simulink model "openMHA_test_FFT_to_gain"  (R2020b)
settings: Solver=VariableStepAuto  StartTime=0.0  StopTime=stop_time  RelTol=1e-3
InitFcn:
  | test_FFT_to_gain_init
StopFcn:
  | test_FFT_to_gain_stop
values from neighbouring files (symbols this model uses):
  accum_delay = max(band_sizes)    [test_FFT_to_gain_init.m]
  accum_delay_memory_size = 2^accum_delay_memory    [test_FFT_to_gain_init.m]
  band_edges = [band_edges mirrored_band_edges]    [test_FFT_to_gain_init.m]
  buf_a = 65.*ones(num_bands,1)    [test_FFT_to_gain_init.m]    (also in test_db_ar_gaintable_init.m)
  buf_r = 65.*ones(num_bands,1)    [test_FFT_to_gain_init.m]    (also in test_db_ar_gaintable_init.m)
  delay_memory_size = 2^system_delay_memory    [test_FFT_to_gain_init.m]
  FFTsize = 256    [test_FFT_to_gain_init.m]    (also in test_db_ar_gaintable_init.m)
  gainapp_dp_memory = log2(num_bands) + 1    [test_FFT_to_gain_init.m]
  num_bands = 8    [test_FFT_to_gain_init.m]    (also in test_db_ar_gaintable_init.m = 2)
  num_bins = FFTsize/2 + 1    (= 129)    [test_FFT_to_gain_init.m]    (also in test_db_ar_gaintable_init.m)
  system_delay = 70    [calculate_gainapp_test_signals.m]    (also in test_FFT_to_gain_init.m = gain_delay + accum_delay)
  table_length = length(gtdata)    [test_FFT_to_gain_init.m]    (also in test_db_ar_gaintable_init.m)
  X_high = 93    [test_FFT_to_gain_init.m]    (also in test_db_ar_gaintable_init.m)
undefined symbols (not defined in the file or in its folder): xIn
libraries: dspsrcs4 x9, hdlsllib x8, simulink x8, FPGA_Open_Speech_Tools x5
(part 1 of 2)
settings Model: SnapshotBufferSize=20  Creator=t96f346  LastModifiedBy=t96f346

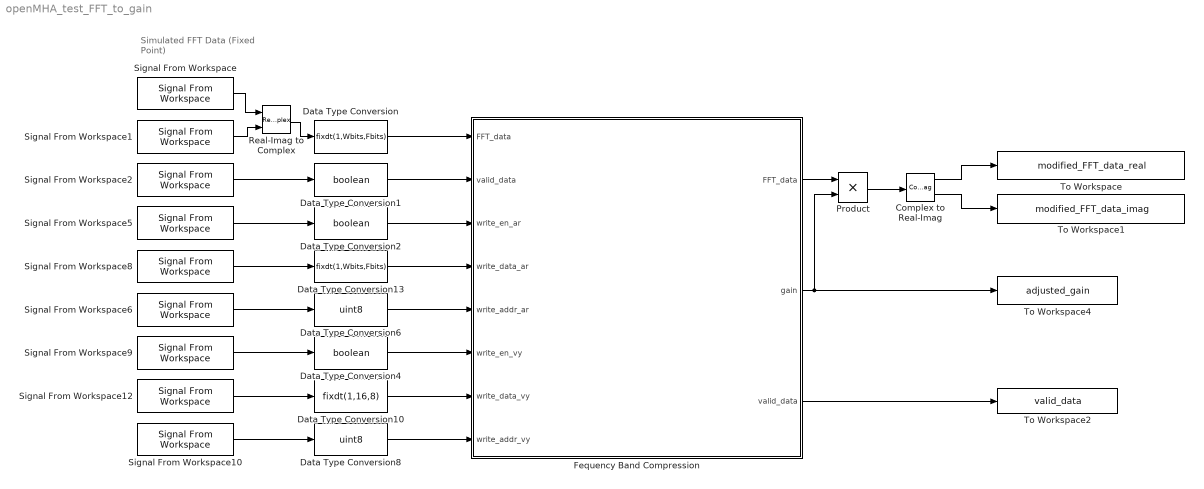
== system openMHA_test_FFT_to_gain ==
  note: Simulated FFT Data
      | (Fixed Point)
  Complex to Real-Imag : ComplexToRealImag
  Data Type Conversion : DataTypeConversion  OutDataTypeStr=fixdt(1,Wbits,Fbits)
  Data Type Conversion1 : DataTypeConversion  OutDataTypeStr=boolean
  Data Type Conversion10 : DataTypeConversion  OutDataTypeStr=fixdt(1,16,8)
  Data Type Conversion13 : DataTypeConversion  OutDataTypeStr=fixdt(1,Wbits,Fbits)
  Data Type Conversion2 : DataTypeConversion  OutDataTypeStr=boolean
  Data Type Conversion4 : DataTypeConversion  OutDataTypeStr=boolean
  Data Type Conversion6 : DataTypeConversion  OutDataTypeStr=uint8
  Data Type Conversion8 : DataTypeConversion  OutDataTypeStr=uint8
  Fequency Band Compression : Subsystem
  Product : Product  OutDataTypeStr=fixdt(1,Wbits,Fbits)
  Real-Imag to Complex : RealImagToComplex
  Signal From Workspace : dspsrcs4/Signal From Workspace  X=FFT_data_real  Ts=1  nsamps=1  OutputAfterFinalValue=Setting to zero  ignoreOrWarnInputAndFrameLengths=off  OutputFrames=off
  Signal From Workspace1 : dspsrcs4/Signal From Workspace  X=FFT_data_imag  Ts=1  nsamps=1  OutputAfterFinalValue=Setting to zero  ignoreOrWarnInputAndFrameLengths=off  OutputFrames=off
  Signal From Workspace10 : dspsrcs4/Signal From Workspace  X=write_addr_vy  Ts=1  nsamps=1  OutputAfterFinalValue=Setting to zero  ignoreOrWarnInputAndFrameLengths=off  OutputFrames=off
  Signal From Workspace12 : dspsrcs4/Signal From Workspace  X=write_data_vy  Ts=1  nsamps=1  OutputAfterFinalValue=Setting to zero  ignoreOrWarnInputAndFrameLengths=off  OutputFrames=off
  Signal From Workspace2 : dspsrcs4/Signal From Workspace  X=valid_data  Ts=1  nsamps=1  OutputAfterFinalValue=Setting to zero  ignoreOrWarnInputAndFrameLengths=off  OutputFrames=off
  Signal From Workspace5 : dspsrcs4/Signal From Workspace  X=write_en_ar  Ts=1  nsamps=1  OutputAfterFinalValue=Setting to zero  ignoreOrWarnInputAndFrameLengths=off  OutputFrames=off
  Signal From Workspace6 : dspsrcs4/Signal From Workspace  X=write_addr_ar  Ts=1  nsamps=1  OutputAfterFinalValue=Setting to zero  ignoreOrWarnInputAndFrameLengths=off  OutputFrames=off
  Signal From Workspace8 : dspsrcs4/Signal From Workspace  X=write_data_ar  Ts=1  nsamps=1  OutputAfterFinalValue=Setting to zero  ignoreOrWarnInputAndFrameLengths=off  OutputFrames=off
  Signal From Workspace9 : dspsrcs4/Signal From Workspace  X=write_en_vy  Ts=1  nsamps=1  OutputAfterFinalValue=Setting to zero  ignoreOrWarnInputAndFrameLengths=off  OutputFrames=off
  To Workspace : ToWorkspace  VariableName=modified_FFT_data_real  SampleTime=-1
      settings: Save2DSignal=2-D array (concatenate along first dimension)
  To Workspace1 : ToWorkspace  VariableName=modified_FFT_data_imag  SampleTime=-1
      settings: Save2DSignal=2-D array (concatenate along first dimension)
  To Workspace2 : ToWorkspace  VariableName=valid_data  SampleTime=-1
      settings: Save2DSignal=2-D array (concatenate along first dimension)
  To Workspace4 : ToWorkspace  VariableName=adjusted_gain  SampleTime=-1
      settings: Save2DSignal=2-D array (concatenate along first dimension)
  wires:
  Real-Imag to Complex/1 -> Data Type Conversion/1
  Signal From Workspace1/1 -> Real-Imag to Complex/2
  Signal From Workspace/1 -> Real-Imag to Complex/1
  Product/1 -> Complex to Real-Imag/1
  Complex to Real-Imag/2 -> To Workspace1/1
  Complex to Real-Imag/1 -> To Workspace/1
  Data Type Conversion/1 -> Fequency Band Compression/1(FFT_data)
  Signal From Workspace2/1 -> Data Type Conversion1/1
  Signal From Workspace12/1 -> Data Type Conversion10/1
  Signal From Workspace8/1 -> Data Type Conversion13/1
  Signal From Workspace10/1 -> Data Type Conversion8/1
  Signal From Workspace9/1 -> Data Type Conversion4/1
  Signal From Workspace6/1 -> Data Type Conversion6/1
  Signal From Workspace5/1 -> Data Type Conversion2/1
  Data Type Conversion2/1 -> Fequency Band Compression/3(write_en_ar)
  Data Type Conversion13/1 -> Fequency Band Compression/4(write_data_ar)
  Data Type Conversion6/1 -> Fequency Band Compression/5(write_addr_ar)
  Data Type Conversion4/1 -> Fequency Band Compression/6(write_en_vy)
  Data Type Conversion10/1 -> Fequency Band Compression/7(write_data_vy)
  Data Type Conversion8/1 -> Fequency Band Compression/8(write_addr_vy)
  Fequency Band Compression/2(gain) -> Product/2, To Workspace4/1
  Data Type Conversion1/1 -> Fequency Band Compression/2(valid_data)
  Fequency Band Compression/1("FFT_data ") -> Product/1
  Fequency Band Compression/3("valid_data ") -> To Workspace2/1

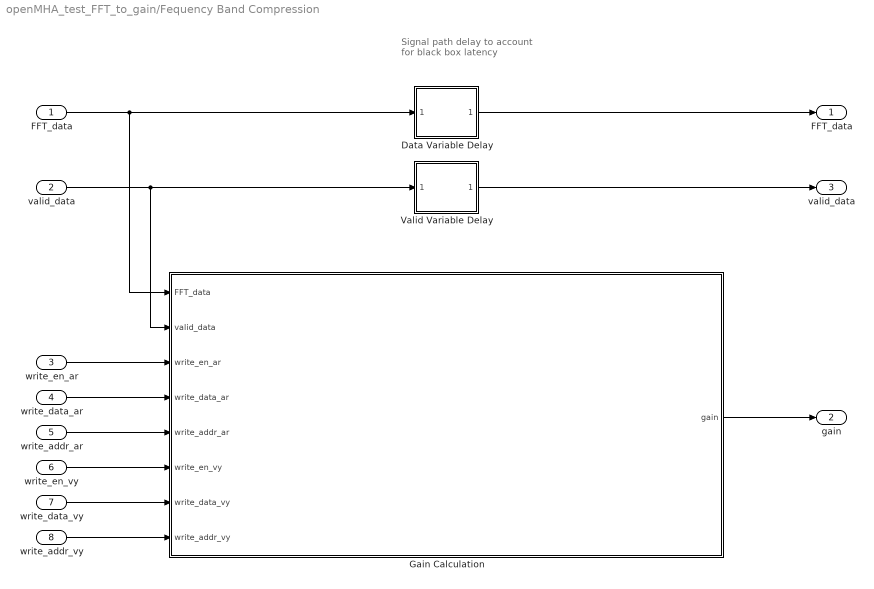
== system openMHA_test_FFT_to_gain/Fequency Band Compression ==
  note: Signal path delay to account for black box latency
  FFT_data : Inport
  valid_data : Inport  Port=2
  write_en_ar : Inport  Port=3
  write_data_ar : Inport  Port=4
  write_addr_ar : Inport  Port=5
  write_en_vy : Inport  Port=6
  write_data_vy : Inport  Port=7
  write_addr_vy : Inport  Port=8
  Data Variable Delay : Subsystem
  Gain Calculation : Subsystem
  Valid Variable Delay : Subsystem
  "FFT_data " : Outport
  gain : Outport  Port=2
  "valid_data " : Outport  Port=3
  wires:
  valid_data/1 -> Gain Calculation/2(valid_data), Valid Variable Delay/1(data_in)
  FFT_data/1 -> Gain Calculation/1(FFT_data), Data Variable Delay/1(data_in)
  Valid Variable Delay/1(rd_dout) -> "valid_data "/1
  Data Variable Delay/1(rd_dout) -> "FFT_data "/1
  write_en_ar/1 -> Gain Calculation/3(write_en_ar)
  write_data_ar/1 -> Gain Calculation/4(write_data_ar)
  write_addr_ar/1 -> Gain Calculation/5(write_addr_ar)
  write_en_vy/1 -> Gain Calculation/6(write_en_vy)
  write_data_vy/1 -> Gain Calculation/7(write_data_vy)
  write_addr_vy/1 -> Gain Calculation/8(write_addr_vy)
  Gain Calculation/1("gain ") -> gain/1

== system openMHA_test_FFT_to_gain/Fequency Band Compression/Data Variable Delay ==
  data_in : Inport
  Constant : Constant  Value=system_delay  OutDataTypeStr=uint8  SampleTime=-1
  Constant2 : Constant  OutDataTypeStr=Inherit: Inherit via back propagation  SampleTime=-1
  integer delay DPRAM : hdlsllib/HDL RAMs/Simple Dual Port RAM  ram_size=system_delay_memory
      settings: SourceProductBaseCode=SL
  read address generator : Subsystem
  write address generator : hdlsllib/Sources/HDL Counter  CountType=Count limited  CountInit=0  CountStep=1  CountMax=delay_memory_size - 1  CountFromType=Initial value  CountFrom=0  CountResetPort=off  CountLoadPort=off  CountEnbPort=off  CountDirPort=off  CountDataType=Unsigned  CountWordLen=system_delay_memory  CountFracLen=0  CountSampTime=-1
  rd_dout : Outport
  wires:
  Constant2/1 -> integer delay DPRAM/3
  write address generator/1 -> integer delay DPRAM/2, read address generator/1(write_addr)
  integer delay DPRAM/1 -> rd_dout/1
  Constant/1 -> read address generator/2(delay)
  data_in/1 -> integer delay DPRAM/1
  read address generator/1(read_addr) -> integer delay DPRAM/4

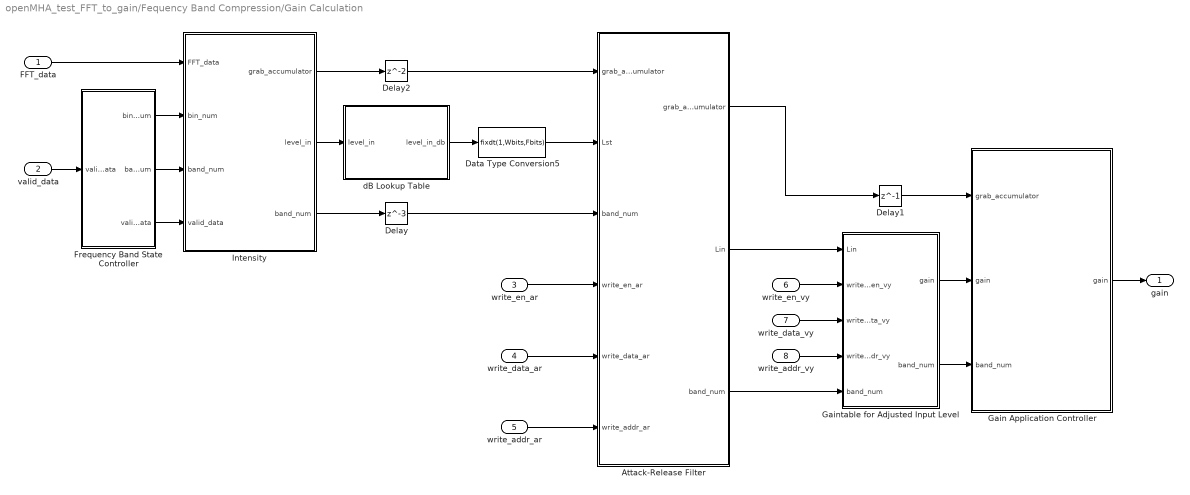
== system openMHA_test_FFT_to_gain/Fequency Band Compression/Gain Calculation ==
  FFT_data : Inport
  valid_data : Inport  Port=2
  write_en_ar : Inport  Port=3
  write_data_ar : Inport  Port=4
  write_addr_ar : Inport  Port=5
  write_en_vy : Inport  Port=6
  write_data_vy : Inport  Port=7
  write_addr_vy : Inport  Port=8
  Attack-Release Filter : Subsystem
  Data Type Conversion5 : DataTypeConversion  OutDataTypeStr=fixdt(1,Wbits,Fbits)
  Delay : Delay  DelayLength=3  InitialCondition=1
  Delay1 : Delay  DelayLength=1  InitialCondition=0
  Delay2 : Delay  InitialCondition=0
  Frequency Band State Controller : Subsystem
  Gain Application Controller : Subsystem
  Gaintable for Adjusted Input Level : Subsystem
  Intensity : Subsystem
  dB Lookup Table : Subsystem
  "gain " : Outport
  wires:
  dB Lookup Table/1(level_in_db) -> Data Type Conversion5/1
  Gaintable for Adjusted Input Level/1(gain) -> Gain Application Controller/2(gain)
  Intensity/1(grab_accumulator) -> Delay2/1
  Delay2/1 -> Attack-Release Filter/1(grab_accumulator)
  write_en_ar/1 -> Attack-Release Filter/4(write_en_ar)
  Frequency Band State Controller/2(band_num) -> Intensity/3(band_num)
  Intensity/3("band_num ") -> Delay/1
  Attack-Release Filter/3("band_num ") -> Gaintable for Adjusted Input Level/5(band_num)
  Delay1/1 -> Gain Application Controller/1(grab_accumulator)
  Delay/1 -> Attack-Release Filter/3(band_num)
  Attack-Release Filter/2(Lin) -> Gaintable for Adjusted Input Level/1(Lin)
  Frequency Band State Controller/1(bin_num) -> Intensity/2(bin_num)
  Gaintable for Adjusted Input Level/2("band_num ") -> Gain Application Controller/3(band_num)
  Data Type Conversion5/1 -> Attack-Release Filter/2(Lst)
  FFT_data/1 -> Intensity/1(FFT_data)
  Intensity/2(level_in) -> dB Lookup Table/1(level_in)
  write_addr_ar/1 -> Attack-Release Filter/6(write_addr_ar)
  valid_data/1 -> Frequency Band State Controller/1(valid_data)
  write_data_ar/1 -> Attack-Release Filter/5(write_data_ar)
  Gain Application Controller/1("gain ") -> "gain "/1
  Attack-Release Filter/1("grab_accumulator ") -> Delay1/1
  write_en_vy/1 -> Gaintable for Adjusted Input Level/2(write_en_vy)
  write_addr_vy/1 -> Gaintable for Adjusted Input Level/4(write_addr_vy)
  write_data_vy/1 -> Gaintable for Adjusted Input Level/3(write_data_vy)
  Frequency Band State Controller/3("valid_data ") -> Intensity/4("valid_data ")

== system openMHA_test_FFT_to_gain/Fequency Band Compression/Valid Variable Delay ==
  data_in : Inport
  Constant : Constant  Value=system_delay  OutDataTypeStr=uint8  SampleTime=-1
  Constant2 : Constant  OutDataTypeStr=Inherit: Inherit via back propagation  SampleTime=-1
  integer delay DPRAM : hdlsllib/HDL RAMs/Simple Dual Port RAM  ram_size=system_delay_memory
      settings: SourceProductBaseCode=SL
  read address generator : Subsystem
  write address generator : hdlsllib/Sources/HDL Counter  CountType=Count limited  CountInit=0  CountStep=1  CountMax=delay_memory_size - 1  CountFromType=Initial value  CountFrom=0  CountResetPort=off  CountLoadPort=off  CountEnbPort=off  CountDirPort=off  CountDataType=Unsigned  CountWordLen=system_delay_memory  CountFracLen=0  CountSampTime=-1
  rd_dout : Outport
  wires:
  Constant2/1 -> integer delay DPRAM/3
  write address generator/1 -> integer delay DPRAM/2, read address generator/1(write_addr)
  integer delay DPRAM/1 -> rd_dout/1
  Constant/1 -> read address generator/2(delay)
  data_in/1 -> integer delay DPRAM/1
  read address generator/1(read_addr) -> integer delay DPRAM/4

== system openMHA_test_FFT_to_gain/Fequency Band Compression/Data Variable Delay/read address generator ==
  note: wrap on overflow is the desired behavior
  write_addr : Inport
  delay : Inport  Port=2
  Constant : Constant  Value=delay_memory_size  SampleTime=-1
  Subtract : Sum  Inputs=-++  OutDataTypeStr=Inherit: Inherit via back propagation
  read_addr : Outport  VectorParamsAs1DForOutWhenUnconnected=off
  wires:
  Subtract/1 -> read_addr/1
  write_addr/1 -> Subtract/2
  delay/1 -> Subtract/1
  Constant/1 -> Subtract/3

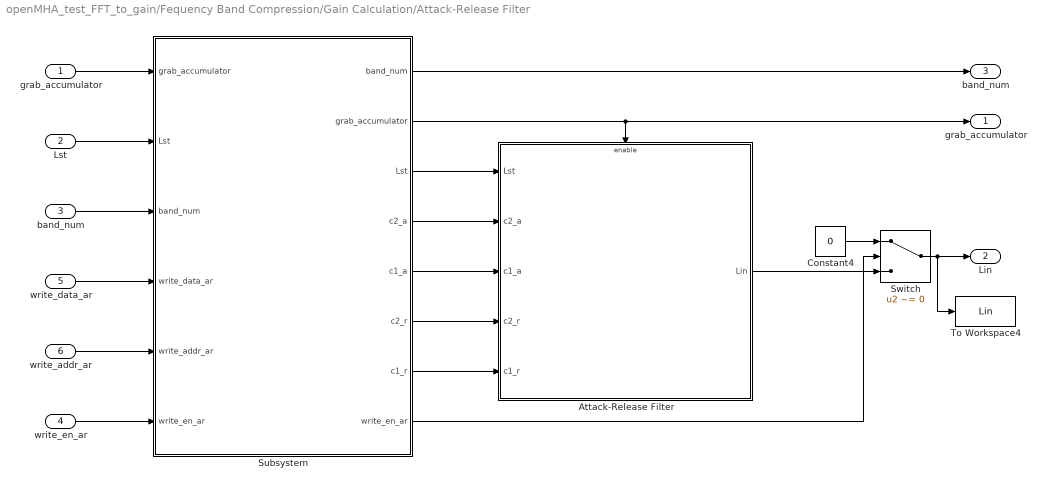
== system openMHA_test_FFT_to_gain/Fequency Band Compression/Gain Calculation/Attack-Release Filter ==
  grab_accumulator : Inport
  Lst : Inport  Port=2
  band_num : Inport  Port=3
  write_en_ar : Inport  Port=4
  write_data_ar : Inport  Port=5
  write_addr_ar : Inport  Port=6
  Attack-Release Filter : Subsystem
  Constant4 : Constant  Value=0  OutDataTypeStr=fixdt(1,Wbits,Fbits)  SampleTime=-1
  Subsystem : Subsystem
  Switch : Switch  Criteria=u2 ~= 0  OutDataTypeStr=fixdt(1,Wbits,Fbits)
  To Workspace4 : ToWorkspace  VariableName=Lin  SampleTime=-1
      settings: Save2DSignal=2-D array (concatenate along first dimension)
  "grab_accumulator " : Outport
  Lin : Outport  Port=2
  "band_num " : Outport  Port=3
  wires:
  Constant4/1 -> Switch/1
  Attack-Release Filter/1(Lin) -> Switch/3
  Switch/1 -> Lin/1, To Workspace4/1
  band_num/1 -> Subsystem/3(band_num)
  Lst/1 -> Subsystem/2(Lst)
  write_data_ar/1 -> Subsystem/4(write_data_ar)
  write_addr_ar/1 -> Subsystem/5(write_addr_ar)
  write_en_ar/1 -> Subsystem/6("write_en_ar ")
  Subsystem/3("Lst ") -> Attack-Release Filter/1(Lst)
  Subsystem/1("band_num ") -> "band_num "/1
  Subsystem/8(write_en_ar) -> Switch/2
  Subsystem/4(c2_a) -> Attack-Release Filter/2(c2_a)
  Subsystem/5(c1_a) -> Attack-Release Filter/3(c1_a)
  Subsystem/6(c2_r) -> Attack-Release Filter/4(c2_r)
  Subsystem/7(c1_r) -> Attack-Release Filter/5(c1_r)
  grab_accumulator/1 -> Subsystem/1(grab_accumulator)
  Subsystem/2("grab_accumulator ") -> "grab_accumulator "/1, Attack-Release Filter/Enable

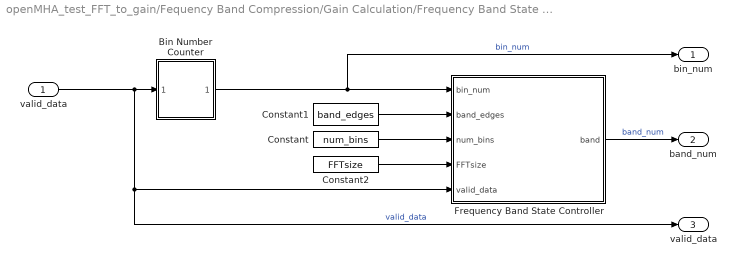
== system openMHA_test_FFT_to_gain/Fequency Band Compression/Gain Calculation/Frequency Band State Controller ==
  valid_data : Inport
  Bin Number Counter : Subsystem
  Constant : Constant  Value=num_bins  SampleTime=-1
  Constant1 : Constant  Value=band_edges  SampleTime=-1
  Constant2 : Constant  Value=FFTsize  SampleTime=-1
  Frequency Band State Controller : MATLAB Function  TreatAsAtomicUnit=on
  bin_num : Outport
  band_num : Outport  Port=2
  "valid_data " : Outport  Port=3
  wires:
  Bin Number Counter/1(bin_num) -> bin_num/1, Frequency Band State Controller/1(bin_num)  "bin_num"
  Constant2/1 -> Frequency Band State Controller/4(FFTsize)
  valid_data/1 -> "valid_data "/1, Frequency Band State Controller/5(valid_data), Bin Number Counter/1(valid_data)  "valid_data"
  Constant/1 -> Frequency Band State Controller/3(num_bins)
  Constant1/1 -> Frequency Band State Controller/2(band_edges)
  Frequency Band State Controller/1(band) -> band_num/1  "band_num"

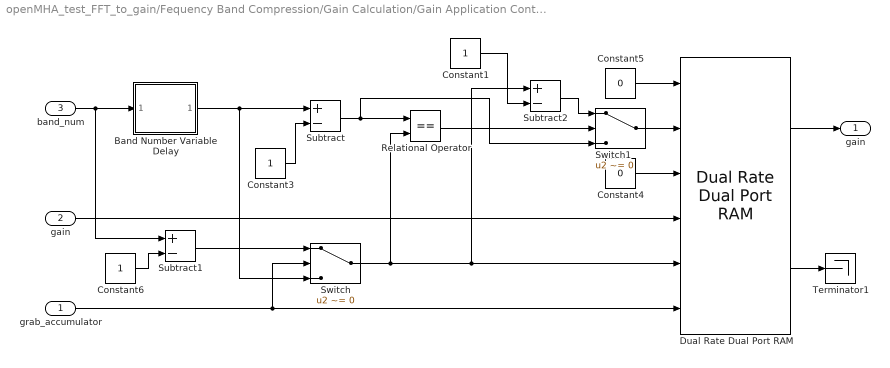
== system openMHA_test_FFT_to_gain/Fequency Band Compression/Gain Calculation/Gain Application Controller ==
  grab_accumulator : Inport
  gain : Inport  Port=2
  band_num : Inport  Port=3
  Band Number Variable Delay : Subsystem
  Constant1 : Constant  SampleTime=-1
  Constant3 : Constant  SampleTime=-1
  Constant4 : Constant  Value=0  OutDataTypeStr=boolean  SampleTime=-1
  Constant5 : Constant  Value=0  OutDataTypeStr=fixdt(1,16,8)  SampleTime=-1
  Constant6 : Constant  SampleTime=-1
  Dual Rate Dual Port RAM : hdlsllib/HDL RAMs/Dual Rate Dual Port RAM  ram_size=gainapp_dp_memory
      settings: SourceProductBaseCode=SL
  Relational Operator : RelationalOperator  Operator===  OutDataTypeStr=boolean  RndMeth=Nearest
  Subtract : Sum  Inputs=+-  OutMin=[0]  OutMax=[2^gainapp_dp_memory-1]  OutDataTypeStr=fixdt(0,gainapp_dp_memory)
  Subtract1 : Sum  Inputs=+-  OutMin=[0]  OutMax=[2^gainapp_dp_memory-1]  OutDataTypeStr=fixdt(0,gainapp_dp_memory)
  Subtract2 : Sum  Inputs=+-  OutMin=[0]  OutMax=[2^gainapp_dp_memory-1]  OutDataTypeStr=fixdt(0,gainapp_dp_memory)
  Switch : Switch  Criteria=u2 ~= 0
  Switch1 : Switch  Criteria=u2 ~= 0
  Terminator1 : Terminator
  "gain " : Outport
  wires:
  Dual Rate Dual Port RAM/1 -> "gain "/1
  Constant5/1 -> Dual Rate Dual Port RAM/1
  Constant6/1 -> Subtract1/2
  Constant3/1 -> Subtract/2
  Constant4/1 -> Dual Rate Dual Port RAM/3
  grab_accumulator/1 -> Dual Rate Dual Port RAM/6, Switch/2
  Subtract1/1 -> Switch/1
  Band Number Variable Delay/1(rd_dout) -> Switch/3, Subtract/1
  Dual Rate Dual Port RAM/2 -> Terminator1/1
  gain/1 -> Dual Rate Dual Port RAM/4
  band_num/1 -> Band Number Variable Delay/1(data_in), Subtract1/1
  Switch/1 -> Relational Operator/2, Dual Rate Dual Port RAM/5, Subtract2/1
  Switch1/1 -> Dual Rate Dual Port RAM/2
  Constant1/1 -> Subtract2/2
  Subtract/1 -> Switch1/3, Relational Operator/1
  Relational Operator/1 -> Switch1/2
  Subtract2/1 -> Switch1/1

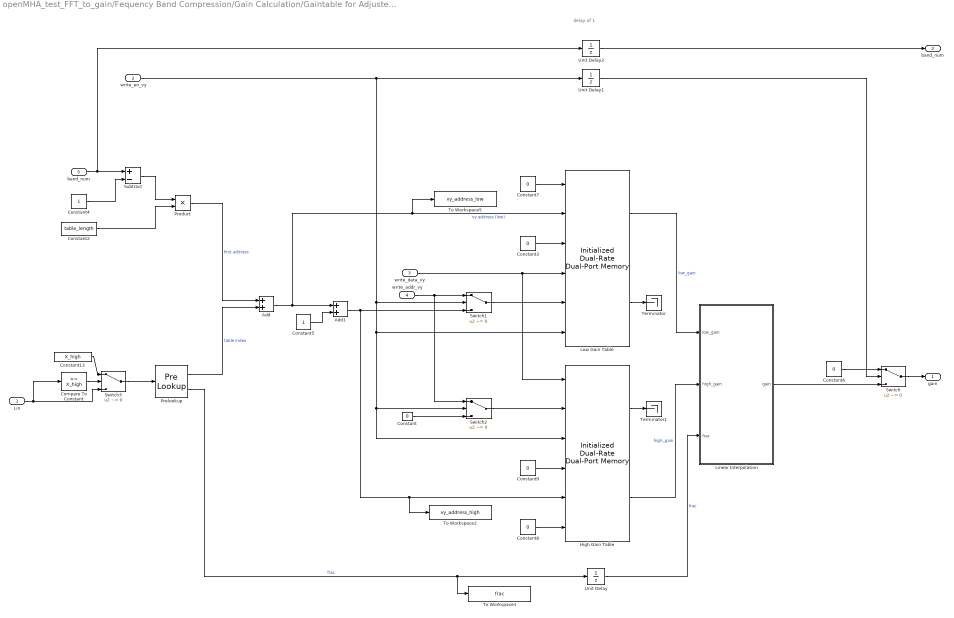
== system openMHA_test_FFT_to_gain/Fequency Band Compression/Gain Calculation/Gaintable for Adjusted Input Level ==
  note: delay of 1
  Lin : Inport
  write_en_vy : Inport  Port=2
  write_data_vy : Inport  Port=3
  write_addr_vy : Inport  Port=4
  band_num : Inport  Port=5
  Add : Sum  OutDataTypeStr=uint8
  Add1 : Sum  OutDataTypeStr=uint8
  Compare To Constant : simulink/Logic and Bit Operations/Compare To Constant  relop=>=  const=X_high  OutDataTypeStr=boolean
  Constant : Constant  Value=0  OutDataTypeStr=uint8  SampleTime=-1
  Constant13 : Constant  Value=X_high  OutDataTypeStr=fixdt(1,Wbits, Fbits)  SampleTime=-1
  Constant2 : Constant  Value=table_length  OutDataTypeStr=uint8  SampleTime=-1
  Constant3 : Constant  Value=0  OutDataTypeStr=boolean  SampleTime=-1
  Constant4 : Constant  OutDataTypeStr=uint8  SampleTime=-1
  Constant5 : Constant  OutDataTypeStr=uint8  SampleTime=-1
  Constant6 : Constant  Value=0  OutDataTypeStr=fixdt(1,16,8)  SampleTime=-1
  Constant7 : Constant  Value=0  OutDataTypeStr=fixdt(1,16,8)  SampleTime=-1
  Constant8 : Constant  Value=0  OutDataTypeStr=boolean  SampleTime=-1
  Constant9 : Constant  Value=0  OutDataTypeStr=fixdt(1,16,8)  SampleTime=-1
  High Gain Table : FPGA_Open_Speech_Tools/Initialized Dual-Rate Dual-Port Memory  ram_size=RAM_size  Table_Init=vy
      settings: SourceProductName=FPGA Open Speech Tools
  Linear Interpolation : Subsystem
  Low Gain Table : FPGA_Open_Speech_Tools/Initialized Dual-Rate Dual-Port Memory  ram_size=RAM_size  Table_Init=vy
      settings: SourceProductName=FPGA Open Speech Tools
  Prelookup : PreLookup  BreakpointsData=input_levels_db  IndexSearchMethod=Evenly spaced points  UseLastBreakpoint=on  DiagnosticForOutOfRangeInput=Error  IndexDataTypeStr=uint8
  Product : Product  OutDataTypeStr=Inherit: Same as first input
  Subtract : Sum  Inputs=+-
  Switch : Switch  Criteria=u2 ~= 0  OutDataTypeStr=fixdt(1,16,8)
  Switch1 : Switch  Criteria=u2 ~= 0
  Switch2 : Switch  Criteria=u2 ~= 0
  Switch3 : Switch  Criteria=u2 ~= 0
  Terminator : Terminator
  Terminator1 : Terminator
  To Workspace1 : ToWorkspace  VariableName=frac  SampleTime=-1
      settings: Save2DSignal=2-D array (concatenate along first dimension)
  To Workspace2 : ToWorkspace  VariableName=vy_address_high  SampleTime=-1
      settings: Save2DSignal=2-D array (concatenate along first dimension)
  To Workspace5 : ToWorkspace  VariableName=vy_address_low  SampleTime=-1
      settings: Save2DSignal=2-D array (concatenate along first dimension)
  Unit Delay : UnitDelay  SampleTime=-1  HasFrameUpgradeWarning=on
  Unit Delay1 : UnitDelay  InitialCondition=1  SampleTime=-1  HasFrameUpgradeWarning=on
  Unit Delay2 : UnitDelay  InitialCondition=1  SampleTime=-1  HasFrameUpgradeWarning=on
  gain : Outport
  "band_num " : Outport  Port=2
  wires:
  Unit Delay/1 -> Linear Interpolation/3(frac)  "frac"
  Unit Delay1/1 -> Switch/2
  Compare To Constant/1 -> Switch3/2
  Switch/1 -> gain/1
  band_num/1 -> Unit Delay2/1, Subtract/1
  Constant6/1 -> Switch/1
  Add/1 -> To Workspace5/1, Low Gain Table/2, Add1/1  "vy address (low)"
  Linear Interpolation/1(gain) -> Switch/3
  write_en_vy/1 -> Switch1/2, High Gain Table/3, Switch2/2, Low Gain Table/6, Unit Delay1/1
  Constant5/1 -> Add1/2
  Prelookup/1 -> Add/2  "table index"
  Constant13/1 -> Switch3/1
  Add1/1 -> To Workspace2/1, High Gain Table/5, Switch1/3
  Low Gain Table/1 -> Linear Interpolation/1(low_gain)  "low_gain"
  Constant4/1 -> Subtract/2
  Prelookup/2 -> To Workspace1/1, Unit Delay/1  "frac"
  Product/1 -> Add/1  "first address"
  Subtract/1 -> Product/1
  Lin/1 -> Compare To Constant/1, Switch3/3
  Constant2/1 -> Product/2
  Switch3/1 -> Prelookup/1
  Unit Delay2/1 -> "band_num "/1
  Low Gain Table/2 -> Terminator/1
  High Gain Table/1 -> Terminator1/1
  Constant8/1 -> High Gain Table/6
  Constant9/1 -> High Gain Table/4
  write_data_vy/1 -> High Gain Table/1, Low Gain Table/4
  write_addr_vy/1 -> Switch2/1, Switch1/1
  Constant7/1 -> Low Gain Table/1
  Constant3/1 -> Low Gain Table/3
  Switch1/1 -> Low Gain Table/5
  Switch2/1 -> High Gain Table/2
  Constant/1 -> Switch2/3
  High Gain Table/2 -> Linear Interpolation/2(high_gain)  "high_gain"

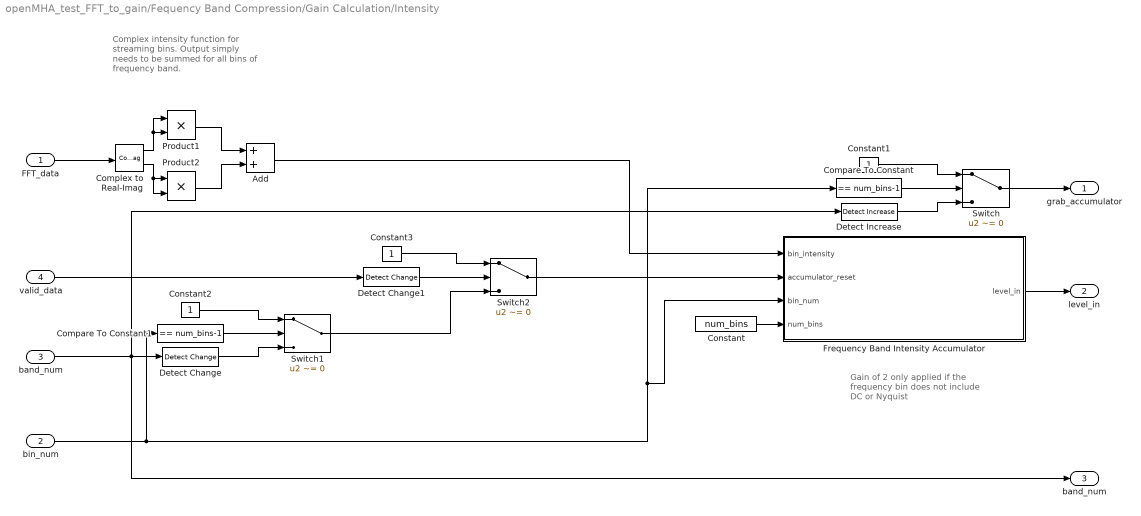
== system openMHA_test_FFT_to_gain/Fequency Band Compression/Gain Calculation/Intensity ==
  note: Complex intensity function for streaming bins. Output simply needs to be summed for all bins of frequency band.
  note: Gain of 2 only applied if the frequency bin does not include DC or Nyquist
  FFT_data : Inport
  bin_num : Inport  Port=2
  band_num : Inport  Port=3
  "valid_data " : Inport  Port=4
  Add : Sum  OutDataTypeStr=fixdt(1,Wbits,Fbits)
  Compare To Constant : simulink/Logic and Bit Operations/Compare To Constant  relop===  const=num_bins-1  OutDataTypeStr=boolean
  Compare To Constant1 : simulink/Logic and Bit Operations/Compare To Constant  relop===  const=num_bins-1  OutDataTypeStr=boolean
  Complex to Real-Imag : ComplexToRealImag
  Constant : Constant  Value=num_bins  OutDataTypeStr=uint8  SampleTime=-1
  Constant1 : Constant  OutDataTypeStr=boolean  SampleTime=-1
  Constant2 : Constant  OutDataTypeStr=boolean  SampleTime=-1
  Constant3 : Constant  OutDataTypeStr=boolean  SampleTime=-1
  Detect Change : simulink/Logic and Bit Operations/Detect Change  vinit=1  OutDataTypeStr=boolean
  Detect Change1 : simulink/Logic and Bit Operations/Detect Change  vinit=1  OutDataTypeStr=boolean
  Detect Increase : simulink/Logic and Bit Operations/Detect Increase  vinit=1  OutDataTypeStr=boolean
  Frequency Band Intensity Accumulator : MATLAB Function  TreatAsAtomicUnit=on
  Product1 : Product  OutDataTypeStr=fixdt(1,Wbits,Fbits)
  Product2 : Product  OutDataTypeStr=fixdt(1,Wbits,Fbits)
  Switch : Switch  Criteria=u2 ~= 0
  Switch1 : Switch  Criteria=u2 ~= 0
  Switch2 : Switch  Criteria=u2 ~= 0
  grab_accumulator : Outport  VectorParamsAs1DForOutWhenUnconnected=off
  level_in : Outport  Port=2
  "band_num " : Outport  Port=3
  wires:
  Product2/1 -> Add/2
  Complex to Real-Imag/1 -> Product1/1, Product1/2
  Complex to Real-Imag/2 -> Product2/2, Product2/1
  Product1/1 -> Add/1
  Add/1 -> Frequency Band Intensity Accumulator/1(bin_intensity)
  FFT_data/1 -> Complex to Real-Imag/1
  Frequency Band Intensity Accumulator/1(level_in) -> level_in/1
  Detect Increase/1 -> Switch/3
  Constant/1 -> Frequency Band Intensity Accumulator/4(num_bins)
  Compare To Constant/1 -> Switch/2
  bin_num/1 -> Compare To Constant1/1, Frequency Band Intensity Accumulator/3(bin_num), Compare To Constant/1
  Constant1/1 -> Switch/1
  Switch/1 -> grab_accumulator/1
  band_num/1 -> "band_num "/1, Detect Increase/1, Detect Change/1
  Constant2/1 -> Switch1/1
  Compare To Constant1/1 -> Switch1/2
  Detect Change/1 -> Switch1/3
  Switch1/1 -> Switch2/3
  "valid_data "/1 -> Detect Change1/1
  Constant3/1 -> Switch2/1
  Detect Change1/1 -> Switch2/2
  Switch2/1 -> Frequency Band Intensity Accumulator/2(accumulator_reset)

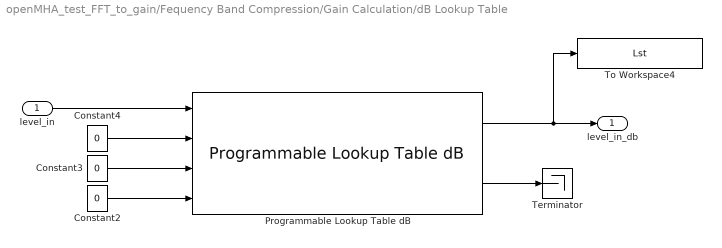
== system openMHA_test_FFT_to_gain/Fequency Band Compression/Gain Calculation/dB Lookup Table ==
  level_in : Inport
  Constant2 : Constant  Value=0  OutDataTypeStr=boolean  SampleTime=-1
  Constant3 : Constant  Value=0  OutDataTypeStr=uint16  SampleTime=-1
  Constant4 : Constant  Value=0  OutDataTypeStr=fixdt(1,40,32)  SampleTime=-1
  Programmable Lookup Table dB : FPGA_Open_Speech_Tools/Programmable Lookup Table dB  tableFnParam=10.*log10(2500000000.*xIn)  SAVE_TABLE=off  maxInput=1  floorParam=2^-31  errorParam=1  ERR_DIAG=on  PLOT_TABLE=off  nBitsParam=5  mBitsParam=4  IGOTTHIS=off  W_bits=40  F_bits=37  tableInit=0  binaryOffset=0
      link override High_LUT/ram_data: InitialCondition=55.36
      link override Linear_Approximation/Unit Delay: InitialCondition=65
      link override LogAddressing/Delay1: InitialCondition=13
      link override LogAddressing/Delay2: InitialCondition=0.0001265
      link override Low_LUT/ram_data: InitialCondition=54.85
      link override Unit Delay1: InitialCondition=0.0001265
      link override Unit Delay2: InitialCondition=0.0001265
      link override Unit Delay3: InitialCondition=144
      settings: SourceProductName=FPGA Open Speech Tools
  Terminator : Terminator
  To Workspace4 : ToWorkspace  VariableName=Lst  SampleTime=-1
      settings: Save2DSignal=2-D array (concatenate along first dimension)
  level_in_db : Outport
  wires:
  Programmable Lookup Table dB/2 -> Terminator/1
  level_in/1 -> Programmable Lookup Table dB/1
  Programmable Lookup Table dB/1 -> To Workspace4/1, level_in_db/1
  Constant4/1 -> Programmable Lookup Table dB/2
  Constant3/1 -> Programmable Lookup Table dB/3
  Constant2/1 -> Programmable Lookup Table dB/4

== system openMHA_test_FFT_to_gain/Fequency Band Compression/Valid Variable Delay/read address generator ==
  note: wrap on overflow is the desired behavior
  write_addr : Inport
  delay : Inport  Port=2
  Constant : Constant  Value=delay_memory_size  SampleTime=-1
  Subtract : Sum  Inputs=-++  OutDataTypeStr=Inherit: Inherit via back propagation
  read_addr : Outport  VectorParamsAs1DForOutWhenUnconnected=off
  wires:
  Subtract/1 -> read_addr/1
  write_addr/1 -> Subtract/2
  delay/1 -> Subtract/1
  Constant/1 -> Subtract/3

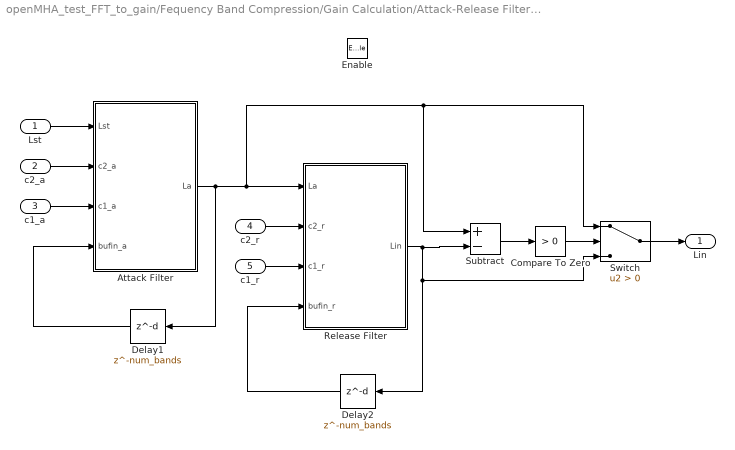
== system openMHA_test_FFT_to_gain/Fequency Band Compression/Gain Calculation/Attack-Release Filter/Attack-Release Filter ==
  Lst : Inport
  c2_a : Inport  Port=2
  c1_a : Inport  Port=3
  c2_r : Inport  Port=4
  c1_r : Inport  Port=5
  Enable : EnablePort
  Attack Filter : Subsystem  TreatAsAtomicUnit=on
  Compare To Zero : simulink/Logic and Bit Operations/Compare To Zero  relop=>  OutDataTypeStr=boolean
  Delay1 : Delay  DelayLength=num_bands  InitialCondition=buf_a  UseCircularBuffer=on
  Delay2 : Delay  DelayLength=num_bands  InitialCondition=buf_r  UseCircularBuffer=on
  Release Filter : Subsystem  TreatAsAtomicUnit=on
  Subtract : Sum  Inputs=+-  OutDataTypeStr=fixdt(0,Wbits,Fbits)
  Switch : Switch  Criteria=u2 > Threshold  OutDataTypeStr=fixdt(0,Wbits,Fbits)
  Lin : Outport  InitialOutput=[buf_r(1,1)]  VectorParamsAs1DForOutWhenUnconnected=off
  wires:
  Lst/1 -> Attack Filter/1(Lst)
  c2_a/1 -> Attack Filter/2(c2_a)
  c1_a/1 -> Attack Filter/3(c1_a)
  Delay1/1 -> Attack Filter/4(bufin_a)
  c2_r/1 -> Release Filter/2(c2_r)
  c1_r/1 -> Release Filter/3(c1_r)
  Delay2/1 -> Release Filter/4(bufin_r)
  Attack Filter/1(La) -> Delay1/1, Switch/1, Subtract/1, Release Filter/1(La)
  Compare To Zero/1 -> Switch/2
  Release Filter/1(Lin) -> Subtract/2, Delay2/1, Switch/3
  Subtract/1 -> Compare To Zero/1
  Switch/1 -> Lin/1

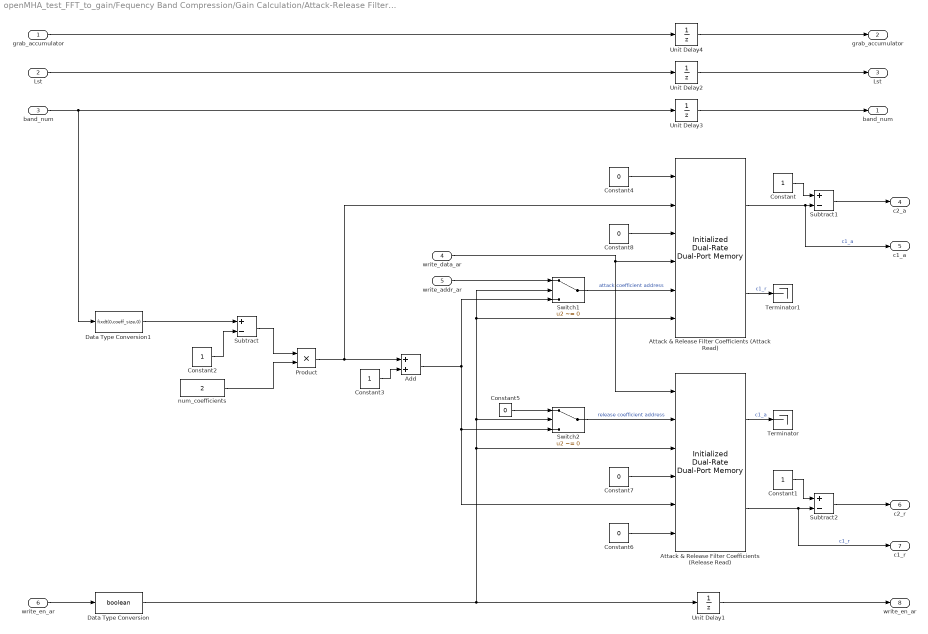
== system openMHA_test_FFT_to_gain/Fequency Band Compression/Gain Calculation/Attack-Release Filter/Subsystem ==
  grab_accumulator : Inport
  Lst : Inport  Port=2
  band_num : Inport  Port=3
  write_data_ar : Inport  Port=4
  write_addr_ar : Inport  Port=5
  "write_en_ar " : Inport  Port=6
  Add : Sum
  Attack & Release Filter Coefficients (Attack Read) : FPGA_Open_Speech_Tools/Initialized Dual-Rate Dual-Port Memory  ram_size=coeff_size  Table_Init=ar_coeffs
      settings: SourceProductName=FPGA Open Speech Tools
  Attack & Release Filter Coefficients (Release Read) : FPGA_Open_Speech_Tools/Initialized Dual-Rate Dual-Port Memory  ram_size=coeff_size  Table_Init=ar_coeffs
      settings: SourceProductName=FPGA Open Speech Tools
  Constant : Constant  OutDataTypeStr=fixdt(1,Wbits,Fbits)  SampleTime=-1
  Constant1 : Constant  OutDataTypeStr=fixdt(1,Wbits,Fbits)  SampleTime=-1
  Constant2 : Constant  OutDataTypeStr=fixdt(0,coeff_size,0)  SampleTime=-1
  Constant3 : Constant  OutDataTypeStr=uint8  SampleTime=-1
  Constant4 : Constant  Value=0  OutDataTypeStr=fixdt(1,Wbits,Fbits)  SampleTime=-1
  Constant5 : Constant  Value=0  OutDataTypeStr=uint8  SampleTime=-1
  Constant6 : Constant  Value=0  OutDataTypeStr=boolean  SampleTime=-1
  Constant7 : Constant  Value=0  OutDataTypeStr=fixdt(1,Wbits,Fbits)  SampleTime=-1
  Constant8 : Constant  Value=0  OutDataTypeStr=boolean  SampleTime=-1
  Data Type Conversion : DataTypeConversion  OutDataTypeStr=boolean
  Data Type Conversion1 : DataTypeConversion  OutDataTypeStr=fixdt(0,coeff_size,0)
  Product : Product  OutDataTypeStr=fixdt(0,coeff_size,0)
  Subtract : Sum  Inputs=+-  OutDataTypeStr=fixdt(0,coeff_size,0)
  Subtract1 : Sum  Inputs=+-  OutDataTypeStr=fixdt(1,Wbits,Fbits)
  Subtract2 : Sum  Inputs=+-  OutDataTypeStr=fixdt(1,Wbits,Fbits)
  Switch1 : Switch  Criteria=u2 ~= 0  OutDataTypeStr=Inherit: Inherit via back propagation
  Switch2 : Switch  Criteria=u2 ~= 0  OutDataTypeStr=uint8
  Terminator : Terminator
  Terminator1 : Terminator
  Unit Delay1 : UnitDelay  SampleTime=-1  HasFrameUpgradeWarning=on
  Unit Delay2 : UnitDelay  InitialCondition=65  SampleTime=-1  HasFrameUpgradeWarning=on
  Unit Delay3 : UnitDelay  InitialCondition=1  SampleTime=-1  HasFrameUpgradeWarning=on
  Unit Delay4 : UnitDelay  SampleTime=-1  HasFrameUpgradeWarning=on
  num_coefficients : Constant  Value=2  OutDataTypeStr=uint8  SampleTime=-1
  "band_num " : Outport
  "grab_accumulator " : Outport  Port=2
  "Lst " : Outport  Port=3
  c2_a : Outport  Port=4
  c1_a : Outport  Port=5
  c2_r : Outport  Port=6
  c1_r : Outport  Port=7
  write_en_ar : Outport  Port=8
  wires:
  num_coefficients/1 -> Product/2
  Data Type Conversion1/1 -> Subtract/1
  Data Type Conversion/1 -> Attack & Release Filter Coefficients (Attack Read)/6, Switch1/2, Switch2/2, Attack & Release Filter Coefficients (Release Read)/3, Unit Delay1/1
  Subtract/1 -> Product/1
  Constant3/1 -> Add/2
  Attack & Release Filter Coefficients (Release Read)/2 -> Subtract2/2, c1_r/1  "c1_r"
  Product/1 -> Attack & Release Filter Coefficients (Attack Read)/2, Add/1
  Constant2/1 -> Subtract/2
  Constant1/1 -> Subtract2/1
  Unit Delay2/1 -> "Lst "/1
  Constant5/1 -> Switch2/1
  Unit Delay1/1 -> write_en_ar/1
  Constant7/1 -> Attack & Release Filter Coefficients (Release Read)/4
  Add/1 -> Switch1/3, Attack & Release Filter Coefficients (Release Read)/5, Switch2/3
  Constant6/1 -> Attack & Release Filter Coefficients (Release Read)/6
  Lst/1 -> Unit Delay2/1
  Switch1/1 -> Attack & Release Filter Coefficients (Attack Read)/5  "attack coefficient address"
  Switch2/1 -> Attack & Release Filter Coefficients (Release Read)/2  "release coefficient address"
  Unit Delay3/1 -> "band_num "/1
  band_num/1 -> Unit Delay3/1, Data Type Conversion1/1
  Subtract2/1 -> c2_r/1
  write_addr_ar/1 -> Switch1/1
  "write_en_ar "/1 -> Data Type Conversion/1
  write_data_ar/1 -> Attack & Release Filter Coefficients (Release Read)/1, Attack & Release Filter Coefficients (Attack Read)/4
  grab_accumulator/1 -> Unit Delay4/1
  Unit Delay4/1 -> "grab_accumulator "/1
  Constant8/1 -> Attack & Release Filter Coefficients (Attack Read)/3
  Constant4/1 -> Attack & Release Filter Coefficients (Attack Read)/1
  Attack & Release Filter Coefficients (Attack Read)/1 -> c1_a/1, Subtract1/2  "c1_a"
  Constant/1 -> Subtract1/1
  Subtract1/1 -> c2_a/1
  Attack & Release Filter Coefficients (Release Read)/1 -> Terminator/1  "c1_a"
  Attack & Release Filter Coefficients (Attack Read)/2 -> Terminator1/1  "c1_r"

== system openMHA_test_FFT_to_gain/Fequency Band Compression/Gain Calculation/Frequency Band State Controller/Bin Number Counter ==
  valid_data : Inport
  Detect Decrease : simulink/Logic and Bit Operations/Detect Decrease  vinit=1  OutDataTypeStr=boolean
  HDL Counter : hdlsllib/Sources/HDL Counter  CountType=Count limited  CountInit=0  CountStep=1  CountMax=FFTsize-1  CountFromType=Initial value  CountFrom=0  CountResetPort=on  CountLoadPort=off  CountEnbPort=on  CountDirPort=off  CountDataType=Unsigned  CountWordLen=log2(FFTsize)  CountFracLen=0  CountSampTime=1
  bin_num : Outport
  wires:
  valid_data/1 -> HDL Counter/2, Detect Decrease/1
  HDL Counter/1 -> bin_num/1
  Detect Decrease/1 -> HDL Counter/1

== system openMHA_test_FFT_to_gain/Fequency Band Compression/Gain Calculation/Gain Application Controller/Band Number Variable Delay ==
  data_in : Inport
  Constant : Constant  Value=accum_delay  OutDataTypeStr=uint8  SampleTime=-1
  Constant2 : Constant  OutDataTypeStr=Inherit: Inherit via back propagation  SampleTime=-1
  integer delay DPRAM : hdlsllib/HDL RAMs/Simple Dual Port RAM  ram_size=accum_delay_memory
      settings: SourceProductBaseCode=SL
  read address generator : Subsystem
  write address generator : hdlsllib/Sources/HDL Counter  CountType=Count limited  CountInit=0  CountStep=1  CountMax=accum_delay_memory_size-1  CountFromType=Initial value  CountFrom=0  CountResetPort=off  CountLoadPort=off  CountEnbPort=off  CountDirPort=off  CountDataType=Unsigned  CountWordLen=accum_delay_memory  CountFracLen=0  CountSampTime=-1
  rd_dout : Outport
  wires:
  Constant2/1 -> integer delay DPRAM/3
  write address generator/1 -> integer delay DPRAM/2, read address generator/1(write_addr)
  integer delay DPRAM/1 -> rd_dout/1
  Constant/1 -> read address generator/2(delay)
  data_in/1 -> integer delay DPRAM/1
  read address generator/1(read_addr) -> integer delay DPRAM/4

== system openMHA_test_FFT_to_gain/Fequency Band Compression/Gain Calculation/Gaintable for Adjusted Input Level/Linear Interpolation ==
  low_gain : Inport
  high_gain : Inport  Port=2
  frac : Inport  Port=3
  Add : Sum
  Product : Product  OutDataTypeStr=Inherit: Same as first input
  Subtract : Sum  Inputs=-+
  gain : Outport
  wires:
  high_gain/1 -> Subtract/2
  low_gain/1 -> Add/1, Subtract/1
  Subtract/1 -> Product/1
  frac/1 -> Product/2
  Product/1 -> Add/2
  Add/1 -> gain/1

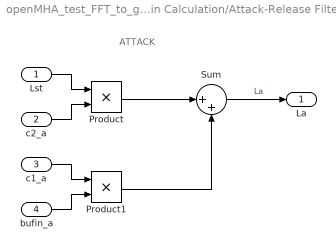
== system openMHA_test_FFT_to_gain/Fequency Band Compression/Gain Calculation/Attack-Release Filter/Attack-Release Filter/Attack Filter ==
  note: ATTACK
  Lst : Inport
  c2_a : Inport  Port=2
  c1_a : Inport  Port=3
  bufin_a : Inport  Port=4
  Product : Product  OutDataTypeStr=fixdt(0,Wbits,Fbits)
  Product1 : Product  OutDataTypeStr=fixdt(0,Wbits,Fbits)
  Sum : Sum  Inputs=|++  OutDataTypeStr=fixdt(0,Wbits,Fbits)
  La : Outport  InitialOutput=0  VectorParamsAs1DForOutWhenUnconnected=off
  wires:
  Lst/1 -> Product/1
  Product/1 -> Sum/1
  Sum/1 -> La/1  "La"
  bufin_a/1 -> Product1/2
  Product1/1 -> Sum/2
  c2_a/1 -> Product/2
  c1_a/1 -> Product1/1

== system openMHA_test_FFT_to_gain/Fequency Band Compression/Gain Calculation/Attack-Release Filter/Attack-Release Filter/Release Filter ==
  note: RELEASE
  La : Inport
  c2_r : Inport  Port=2
  c1_r : Inport  Port=3
  bufin_r : Inport  Port=4
  Product : Product  OutDataTypeStr=fixdt(0,Wbits,Fbits)
  Product1 : Product  OutDataTypeStr=fixdt(0,Wbits,Fbits)
  Sum : Sum  Inputs=|++  OutDataTypeStr=fixdt(0,Wbits,Fbits)
  Lin : Outport  InitialOutput=0  VectorParamsAs1DForOutWhenUnconnected=off
  wires:
  Sum/1 -> Lin/1  "Lin"
  c2_r/1 -> Product/2
  c1_r/1 -> Product1/1
  La/1 -> Product/1
  Product1/1 -> Sum/2
  Product/1 -> Sum/1
  bufin_r/1 -> Product1/2

== system openMHA_test_FFT_to_gain/Fequency Band Compression/Gain Calculation/Gain Application Controller/Band Number Variable Delay/read address generator ==
  note: wrap on overflow is the desired behavior
  write_addr : Inport
  delay : Inport  Port=2
  Constant : Constant  Value=accum_delay_memory_size  SampleTime=-1
  Subtract : Sum  Inputs=-++  OutDataTypeStr=Inherit: Inherit via back propagation
  read_addr : Outport  VectorParamsAs1DForOutWhenUnconnected=off
  wires:
  Subtract/1 -> read_addr/1
  write_addr/1 -> Subtract/2
  delay/1 -> Subtract/1
  Constant/1 -> Subtract/3
